simulink model "px4_6dof_quadrotor_simscape"  (R2023a)
settings: Solver=FixedStepAuto  StartTime=0.0  StopTime=timespot_spl(end)+2  FixedStep=0.001  MaxStep=1e-2  RelTol=1e-3  AbsTol=1e-3
model workspace (MATLAB code in the model file):
  | load('xy_data_membrane.mat');
undefined symbols (not defined in the file or in its folder): air_rho, battery_capacity, DiscIntNeverNeededParam, drone_leg, filtD_motor, filtSpd_motor, kd_motor, ki_motor, kp_motor, limit_motor, pkgSize, planedepth, qc_motor, qd_area, qd_drag, rad, s, spline_data, spline_yaw, timespot_spl, waypoints, wind_speed, X, Y, Z
libraries: sm_lib x77, nesl_utility x30, fl_lib x13, cstblocks x9, simulink x8, quadcopter_library x6, aerolibconvert2 x4, slpidlib x4, ee_lib x4, sharedtransform x1, batteryecm_lib x1
(part 1 of 4)
CloseFcn:
  | try,close(h1_quadcopter_package_delivery),end
  | clear h1_quadcopter_package_delivery
  | try,close(h2_quadcopter_package_delivery),end
  | clear h2_quadcopter_package_delivery
  | try,close(h3_quadcopter_package_delivery),end
  | clear h3_quadcopter_package_delivery
  | try,close(h4_quadcopter_package_delivery),end
  | clear h4_quadcopter_package_delivery
Description:
  | Quadcopter Package Delivery
  | Copyright 2021-2023 The MathWorks, Inc.
settings Model: VariantFading=off  Creator=tianwang  LastModifiedBy=user
settings SolverCC: AutoScaleAbsTol=off  AlgebraicLoopSolver=TrustRegion  SolverResetMethod=Robust
settings DataIOCC: MaxDataPoints=10000  ReturnWorkspaceOutputs=off  SignalLoggingName=logsout_quadcopter_package_delivery
settings OptimizationCC: ReuseModelBlockBuffer=off
settings DebuggingCC: ParameterPrecisionLossMsg=none  UnconnectedInputMsg=warning  UnconnectedOutputMsg=warning  UnconnectedLineMsg=warning
settings ModelReferenceCC: EnableRefExpFcnMdlSchedulingChecks=on
settings SFSimCC: CustomCodeUndefinedFunction=UseInterfaceOnly
settings RTWCC: DLArmComputeVersion=19.05
settings SimscapeCC: ExplicitSolverDiagnosticOptions=none  SimscapeLogType=all  SimscapeLogSimulationStatistics=on  SimscapeLogToSDI=on  SimscapeLogName=simlog_quadcopter_package_delivery  SimscapeLogLimitData=off  SimscapeLogDataHistory=50000
settings DiagnosticsConfigSet: SimMechanicsConflictingReferenceFrames=none  SimMechanicsRigidlyBoundBlock=none
settings ExplorerConfigSet: InternalSimMechanicsExplorerSettings="<ExplorerConfiguration><canonicalview>default</canonicalview><AnimationSetting><BasePlaybackSpeed>1.0</BasePlaybackSpeed><PlaybackSpeedFactor>2.0</PlaybackSpeedFactor></AnimationSetting><TilePanel><TileInfo><Tiles Columns=\"2\" Count=\"4\" Rows=\"2\"><Column Weight=\"0.5664\"/><Column Weight=\"0.4336\"/><Row Weight=\"0.3531\"/><Row Weight=\"0.6469\"/><Tile Height=\"1\" Width=\"1\" X=\"0\" Y=\"0\"/><Tile Height=\"1\" Width=\"1\" X=\"0\" Y=\"1\"/><Tile Height=\"1\" Width=\"1\" X=\"1\" Y=\"0\"/><Tile Height=\"1\" Width=\"1\" X=\"1\" Y=\"1\"/></Tiles></TileInfo><SceneInfo><SceneViewer><BGColor><R>1</R><G>1</G><B>1</B></BGColor><Camera><DoPerspective>off</DoPerspective><Position><X>3.00027489530859626</X><Y>2.64492473252887361</Y><Z>13.644244441979108</Z></Position><Center><X>3.00027489530859626</X><Y>2.64492473252887361</Y><Z>3.00000062058594352</Z></Center><Up><X>0</X><Y>1</Y><Z>-0</Z></Up><ViewLimDist>1</ViewLimDist><YLim>10.5985457420349132</YLim><XLim>33.4261827248793395</XLim></Camera></SceneViewer><SceneViewer><BGColor><R>1</R><G>1</G><B>1</B></BGColor><Camera><DoPerspective>on</DoPerspective><Position><X>5.02017998369651863</X><Y>7.98844218227809488</Y><Z>3.70518563279751856</Z></Position><Center><X>5.02017998369651863</X><Y>7.98844218227809488</Y><Z>2.70518563279751856</Z></Center><Up><X>0</X><Y>1</Y><Z>0</Z></Up><ViewLimDist>1</ViewLimDist><YLim>0.466307658154998583</YLim><XLim>0.796608916014789226</XLim></Camera></SceneViewer><SceneViewer><BGColor><R>1</R><G>1</G><B>1</B></BGColor><Camera><DoPerspective>on</DoPerspective><Position><X>6.5</X><Y>6.5</Y><Z>1</Z></Position><Center><X>5</X><Y>8</Y><Z>0</Z></Center><Up><X>0</X><Y>0</Y><Z>1</Z></Up><ViewLimDist>1</ViewLimDist><YLim>0.466307658154998583</YLim><XLim>1.12272536155780434</XLim></Camera></SceneViewer><SceneViewer><BGColor><R>1</R><G>1</G><B>1</B></BGColor><Camera><DoPerspective>on</DoPerspective><Position><X>5.52017998369651863</X><Y>6.98844218227809488</Y><Z>3.70518563279751856</Z></Position><Center><X>5.1868466503631856</X><Y>7.65510884894476185</Y><Z>3.0385189661308516</Z></Center><Up><X>-0.298142396999971915</X><Y>0.596284793999944052</Y><Z>0.745355992499929787</Z></Up><ViewLimDist>1</ViewLimDist><YLim>0.466307658154998583</YLim><XLim>0.608142904177144006</XLim></Camera></SceneViewer></SceneInfo></TilePanel><MechEditorPanel><Cameras><Camera><Id>Camera1</Id><Value><Name>FixO Top</Name><NativeCamera><PositionTrackingFeature>Quadcopter.Camera.Cam_FixO_Top.R</PositionTrackingFeature><CenterTrackingFeature>Quadcopter.Camera.Cam_FixO_Top.R</CenterTrackingFeature><UpVectorTrackingFeature>Quadcopter.Camera.Cam_FixO_Top.R</UpVectorTrackingFeature><CenterTrackingOrigin>off</CenterTrackingOrigin><CenterTrackingDirection>+X</CenterTrackingDirection><UpVectorTrackingDirection>+Y</UpVectorTrackingDirection></NativeCamera></Value></Camera><Camera><Id>Camera2</Id><Value><Name>FixO L</Name><NativeCamera><PositionTrackingFeature>Quadcopter.Camera.Cam_FixO_L.R</PositionTrackingFeature><CenterTrackingFeature>Quadcopter.Camera.Cam_FixO_L.R</CenterTrackingFeature><UpVectorTrackingFeature>Quadcopter.Camera.Cam_FixO_L.R</UpVectorTrackingFeature><CenterTrackingOrigin>off</CenterTrackingOrigin><CenterTrackingDirection>+X</CenterTrackingDirection><UpVectorTrackingDirection>+Z</UpVectorTrackingDirection></NativeCamera></Value></Camera><Camera><Id>Camera3</Id><Value><Name>FixO F</Name><NativeCamera><PositionTrackingFeature>Quadcopter.Camera.Cam_FixO_F.R</PositionTrackingFeature><CenterTrackingFeature>Quadcopter.Camera.Cam_FixO_F.R</CenterTrackingFeature><UpVectorTrackingFeature>Quadcopter.Camera.Cam_FixO_F.R</UpVectorTrackingFeature><CenterTrackingOrigin>off</CenterTrackingOrigin><CenterTrackingDirection>+X</CenterTrackingDirection><UpVectorTrackingDirection>+Z</UpVectorTrackingDirection></NativeCamera></Value></Camera><Camera><Id>Camera4</Id><Value><Name>FixO UFL</Name><NativeCamera><PositionTrackingFeature>Quadcopter.Camera.Cam_FixO_UFL.R</PositionTrackingFeature><CenterTrackingFeature>Quadcopter.Camera.Cam_FixO_UFL.R</CenterTrackingFeature><UpVectorTrackingFeature>Quadcopter.Camera.Cam_FixO_UFL.R</UpVectorTrackingFeature><CenterTrackingOrigin>off</CenterTrackingOrigin><CenterTrackingDirection>+X</CenterTrackingDirection><UpVectorTrackingDirection>+Z</UpVectorTrackingDirection></NativeCamera></Value></Camera><Camera><Id>Camera5</Id><Value><Name>Track_Target</Name><NativeCamera><PositionTrackingFeature>Quadcopter.Camera.Cam_Target.R</PositionTrackingFeature><CenterTrackingFeature>Quadcopter.Camera.Transform_Target.F</CenterTrackingFeature><UpVectorTrackingFeature>Quadcopter.Camera.Transform_Target.F</UpVectorTrackingFeature><CenterTrackingOrigin>on</CenterTrackingOrigin><UpVectorTrackingDirection>+Z</UpVectorTrackingDirection></NativeCamera></Value></Camera><Camera><Id>Camera6</Id><Value><Name>Track Body Forward</Name><NativeCamera><PositionTrackingFeature>Quadcopter.Body.Body.Cam_Body_Front.R</PositionTrackingFeature><CenterTrackingFeature>Quadcopter.Body.Body.Cam_Body_Front.R</CenterTrackingFeature><UpVectorTrackingFeature>Quadcopter.Body.Body.Cam_Body_Front.R</UpVectorTrackingFeature><CenterTrackingOrigin>off</CenterTrackingOrigin><CenterTrackingDirection>+X</CenterTrackingDirection><UpVectorTrackingDirection>+Z</UpVectorTrackingDirection></NativeCamera></Value></Camera></Cameras><GfxPanelCameraMap><MapElement CameraMLId=\"Camera1\" GfxPanelIndex=\"1\"/><MapElement CameraMLId=\"Camera5\" GfxPanelIndex=\"2\"/><MapElement CameraMLId=\"Camera4\" GfxPanelIndex=\"3\"/></GfxPanelCameraMap><VideoCreator><PlaybackSpeedRatio>1.0</PlaybackSpeedRatio><FrameRate>60</FrameRate><VideoFormat>MPEG-4</VideoFormat><FrameSize>[1920 1080]</FrameSize></VideoCreator></MechEditorPanel></ExplorerConfiguration>"

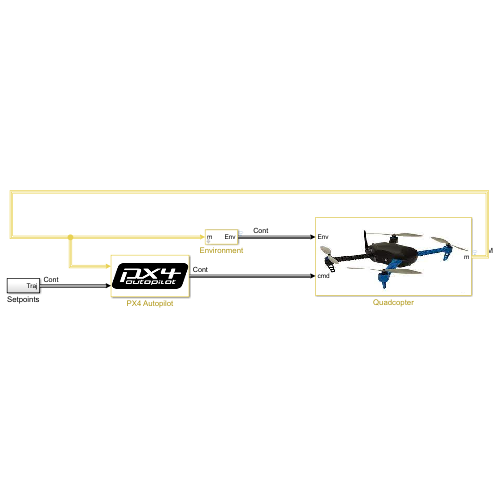
[thumbnail: Simulink's stored preview of the top-level diagram]
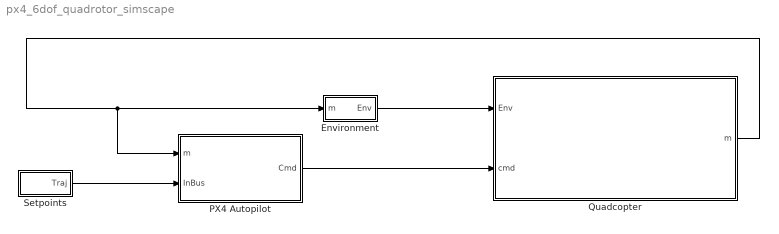
== system px4_6dof_quadrotor_simscape ==
  Environment : Subsystem  mask{wind_speed_mag=wind_speed, height_max_wind=6, height_min_wind=2}
      mask prompts: wind_speed_mag "Wind Speed for Gust (m/s)"; height_max_wind "Lowest Height for Max Wind (m)"; height_min_wind "Maximum Height for Zero Wind (m)"
  PX4 Autopilot : Subsystem
      mask Display:
      | image('C:\Users\user\Desktop\px4_simulink_simulator\docs\px4.png'); % Use "Edit Image" on toolstrip to change.
      | 
      | % port_label('input',1,'m')
      | % port_label('input',2,'Position S.P')
      | %
      | % port_label('output',1,'cmd','texmode','on')
  Quadcopter : Subsystem
      mask Display: image('C:\Users\user\Desktop\px4_simulink_simulator\docs\iris.jpg'); % Use "Edit Image" on toolstrip to change.
  Setpoints : Subsystem
  wires:
  Quadcopter/1(m) -> Environment/1(m), PX4 Autopilot/1(m)
  Setpoints/1(Traj) -> PX4 Autopilot/2(InBus)
  Environment/1(Env) -> Quadcopter/1(Env)
  PX4 Autopilot/1(Cmd) -> Quadcopter/2(cmd)

== system px4_6dof_quadrotor_simscape/Environment ==
  In Bus Element : Inport  PortName=m  Element=Chassis.pz
  Bias Height Min Wind : Bias  Bias=-height_min_wind  SaturateOnIntegerOverflow=off
  Bus Creator2 : BusCreator  Inputs=1
  Constant1 : Constant  Value=0
  Mux1 : Mux  Inputs=3
  Product1 : Product
  Pulse Generator2 : DiscretePulseGenerator  PulseType=Time based  Amplitude=wind_speed_mag  Period=10  PulseWidth=25  PhaseDelay=5
  Pulse Generator3 : DiscretePulseGenerator  PulseType=Time based  Amplitude=wind_speed_mag  Period=10  PulseWidth=25  PhaseDelay=9
  Saturation : Saturate  UpperLimit=height_max_wind-height_min_wind  LowerLimit=0  ZeroCross=off
  "Scale Wind by Height " : Gain  Gain=1/(height_max_wind-height_min_wind)
  Vec to Bus : Subsystem
  Env : Outport
  wires:
  In Bus Element/1 -> Bias Height Min Wind/1
  Bias Height Min Wind/1 -> Saturation/1
  Saturation/1 -> "Scale Wind by Height "/1
  "Scale Wind by Height "/1 -> Product1/1
  Constant1/1 -> Mux1/3  "vz"
  Pulse Generator3/1 -> Mux1/2  "vy"
  Pulse Generator2/1 -> Mux1/1  "vx"
  Mux1/1 -> Product1/2  "wind"
  Product1/1 -> Vec to Bus/1(V)  "wind"
  Vec to Bus/1(B) -> Bus Creator2/1
  Bus Creator2/1 -> Env/1  "Env"

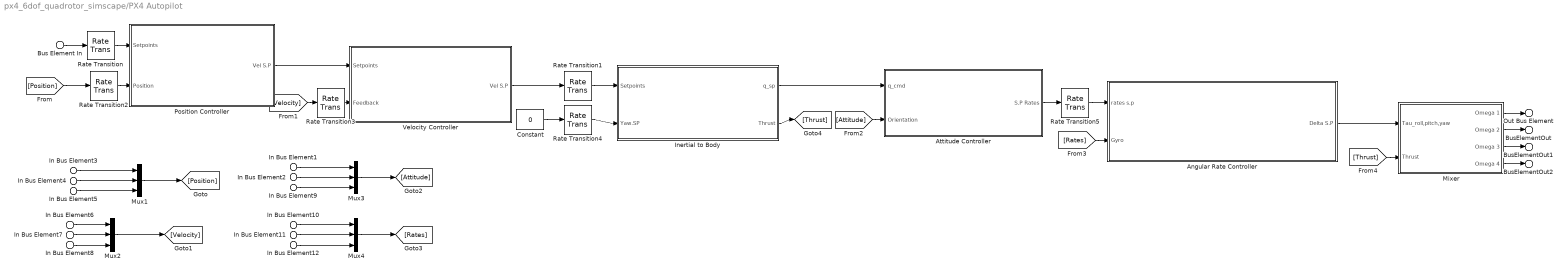
== system px4_6dof_quadrotor_simscape/PX4 Autopilot ==
  In Bus Element3 : Inport  PortName=m  Element=Chassis.px
  In Bus Element4 : Inport  PortName=m  Element=Chassis.py
  In Bus Element5 : Inport  PortName=m  Element=Chassis.pz
  In Bus Element6 : Inport  PortName=m  Element=Chassis.vx
  In Bus Element7 : Inport  PortName=m  Element=Chassis.vy
  In Bus Element8 : Inport  PortName=m  Element=Chassis.vz
  In Bus Element1 : Inport  PortName=m  Element=Chassis.roll
  In Bus Element2 : Inport  PortName=m  Element=Chassis.pitch
  In Bus Element9 : Inport  PortName=m  Element=Chassis.yaw
  In Bus Element10 : Inport  PortName=m  Element=Chassis.nRoll
  In Bus Element11 : Inport  PortName=m  Element=Chassis.nPitch
  In Bus Element12 : Inport  PortName=m  Element=Chassis.nYaw
  Bus Element In : Inport  Port=2  PortName=InBus  Element=pos
  Angular Rate Controller : Subsystem  mask{MC_ROLLRATE_K=1, MC_ROLLRATE_P=0.044, MC_ROLLRATE_I=0.05, MC_ROLLRATE_D=0.0012, MC_RR_INT_LIM=101, MC_PITCHRATE_K=1, MC_PITCHRATE_P=0.044, MC_PITCHRATE_I=0.05, MC_PITCHRATE_D=0.0012, MC_PR_INT_LIM=100, MC_YAWRATE_K=1, MC_YAWRATE_P=0.044, MC_YAWRATE_I=0.05, MC_YAWRATE_D=0.0012, MC_YR_INT_LIM=100, IMU_DGYRO_CUTOFF=6000, IMU_GYRO_CUTOFF=0}
      mask prompts: MC_ROLLRATE_K "MC_ROLLRATE_K ="; MC_ROLLRATE_P "MC_ROLLRATE_P ="; MC_ROLLRATE_I "MC_ROLLRATE_I ="; MC_ROLLRATE_D "MC_ROLLRATE_D ="; MC_RR_INT_LIM "MC_RR_INT_LIM ="; MC_PITCHRATE_K "MC_PITCHRATE_K ="; MC_PITCHRATE_P "MC_PITCHRATE_P ="; MC_PITCHRATE_I "MC_PITCHRATE_I ="; MC_PITCHRATE_D "MC_PITCHRATE_D ="; MC_PR_INT_LIM "MC_PR_INT_LIM ="; MC_YAWRATE_K "MC_YAWRATE_K ="; MC_YAWRATE_P "MC_YAWRATE_P ="; MC_YAWRATE_I "MC_YAWRATE_I ="; MC_YAWRATE_D "MC_YAWRATE_D ="; MC_YR_INT_LIM "MC_YR_INT_LIM ="; IMU_DGYRO_CUTOFF "IMU_DGYRO_CUTOFF ="; IMU_GYRO_CUTOFF "IMU_GYRO_CUTOFF ="
      mask DialogControl DescTextVar Prompt: Angular rate controller, based on PX4 architecture
      mask DialogControl ROLL Prompt: Roll
      mask DialogControl PITCH Prompt: Pitch
      mask DialogControl YAW Prompt: Yaw
      mask Display:
      | disp('Angular Rate Controller')
      | 
      | port_label('input',1,'RATE S.P','texmode','on')
      | port_label('input',2,'Rates','texmode','on')
      | 
      | port_label('output',1,'\delta_{cmd}','texmode','on')
  Attitude Controller : Subsystem  mask{MC_ROLL_P=4, MC_PITCH_P=4, MC_YAW_P=4, MC_ROLLRATE_MAX=2, MC_PITCHRATE_MAX=2, MC_YAWRATE_MAX=2, MC_ACRO_R_MAX=2, MC_YAW_WEIGHT=0.1, m=0.9}
      mask prompts: MC_ROLL_P "MC_ROLL_P ="; MC_PITCH_P "MC_PITCH_P ="; MC_YAW_P "MC_YAW_P ="; MC_ROLLRATE_MAX "MC_ROLLRATE_MAX ="; MC_PITCHRATE_MAX "MC_PITCHRATE_MAX ="; MC_YAWRATE_MAX "MC_YAWRATE_MAX ="; MC_ACRO_R_MAX "MC_ACRO_R_MAX ="; MC_YAW_WEIGHT "MC_YAW_WEIGHT ="; m "m [kg] ="
      mask DialogControl DescTextVar Prompt: Attitude Controller - based on PX4 architecture
      mask Display:
      | disp('Attitude Controller')
      | 
      | port_label('input',1,'q_{sp}','texmode','on')
      | port_label('input',2,'Attitude')
      | 
      | port_label('output',1,'RATES S.P','texmode','on')
  Constant : Constant  Value=0
  Inertial to Body : Subsystem
      mask DialogControl DescTextVar Prompt: Attitude Controller - based on PX4 architecture
      mask Display:
      | disp('Inertial to Body')
      | 
      | port_label('input',1,'ACCEL. S.P')
      | port_label('input',2,'\psi_{cmd}','texmode','on')
      | 
      | port_label('output',1,'q_{sp}','texmode','on')
      | port_label('output',2,'Thrust_{cmd}','texmode','on')
  Mixer : Subsystem  mask{Ct=7e-6, Cq=1.6e-7, d=0.165}
      mask prompts: Ct "Ct ="; Cq "Cq ="; d "d [m] ="
      mask Display:
      | disp('Mixer')
      | 
      | port_label('input',1,'\delta_{cmd}','texmode','on')
      | port_label('input',2,'Thrust_{cmd}','texmode','on')
      | 
      | port_label('output',1,'\Omega_{1cmd}','texmode','on')
      | port_label('output',2,'\Omega_{2cmd}','texmode','on')
      | port_label('output',3,'\Omega_{3cmd}','texmode','on')
      | port_label('output',4,'\Omega_{4cmd}','texmode','on')
  Mux{1..4} (4 alike) : Mux  Inputs=3
  Position Controller : Subsystem  mask{MPC_XY_P=1, MPC_XY_VEL_MAX=10, MPC_Z_P=1, MPC_Z_VEL_MAX_UP=100, MPC_Z_VEL_MAX_DOWN=-100}
      mask prompts: MPC_XY_P "MPC_XY_P ="; MPC_XY_VEL_MAX "MPC_XY_VEL_MAX ="; MPC_Z_P "MPC_Z_P ="; MPC_Z_VEL_MAX_UP "MPC_Z_VEL_MAX_UP ="; MPC_Z_VEL_MAX_DOWN "MPC_Z_VEL_MAX_DOWN ="
      mask DialogControl DescTextVar Prompt: Position Controller - based on PX4 architecture
      mask Display:
      | disp('Position Controller')
      | 
      | port_label('input',1,'POS. S.P')
      | port_label('input',2,'Position')
      | 
      | port_label('output',1,'VEL. S.P','texmode','on')
  Rate Transition : RateTransition  OutPortSampleTime=1/50
  Rate Transition1 : RateTransition  OutPortSampleTime=1/1000
  Rate Transition2 : RateTransition  OutPortSampleTime=1/50
  Rate Transition3 : RateTransition  OutPortSampleTime=1/50
  Rate Transition4 : RateTransition  OutPortSampleTime=1/ 250
  Rate Transition5 : RateTransition  OutPortSampleTime=1/1000
  Velocity Controller : Subsystem  mask{MPC_XY_VEL_P_ACC=1, MPC_XY_VEL_I_ACC=0.1, MPC_XY_VEL_D_ACC=0.05, MPC_Z_VEL_P_ACC=1, MPC_Z_VEL_I_ACC=0.1, MPC_Z_VEL_D_ACC=0.05, MPC_VELD_LP=0, MPC_TILTMAX_AIR=1000, MPC_THR_MAX=10000}
      mask prompts: MPC_XY_VEL_P_ACC "MPC_XY_VEL_P_ACC ="; MPC_XY_VEL_I_ACC "MPC_XY_VEL_I_ACC ="; MPC_XY_VEL_D_ACC "MPC_XY_VEL_D_ACC ="; MPC_Z_VEL_P_ACC "MPC_Z_VEL_P_ACC ="; MPC_Z_VEL_I_ACC "MPC_Z_VEL_I_ACC ="; MPC_Z_VEL_D_ACC "MPC_Z_VEL_D_ACC ="; MPC_VELD_LP "MPC_VELD_LP ="; MPC_TILTMAX_AIR "MPC_TILTMAX_AIR ="; MPC_THR_MAX "MPC_THR_MAX ="
      mask DialogControl DescTextVar Prompt: Velocity Controller - based on PX4 architecture
      mask DialogControl Container3 Prompt: XY -  Velocity
      mask DialogControl Container4 Prompt: Z - Velocity
      mask DialogControl Container5 Prompt: General Parameters
      mask Display:
      | disp('Velocity Controller')
      | 
      | port_label('input',1,'VEL. S.P')
      | port_label('input',2,'Velocity')
      | 
      | port_label('output',1,'ACCEL. S.P','texmode','on')
  Out Bus Element : Outport  PortName=Cmd  Element=w1
  BusElementOut : Outport  PortName=Cmd  Element=w2
  BusElementOut1 : Outport  PortName=Cmd  Element=w3
  BusElementOut2 : Outport  PortName=Cmd  Element=w4
  wires:
  Inertial to Body/1(q_sp) -> Attitude Controller/1(q_cmd)
  Angular Rate Controller/1(Delta S.P) -> Mixer/1(Tau_roll,pitch,yaw)
  Rate Transition4/1 -> Inertial to Body/2(Yaw.SP)
  Velocity Controller/1(Vel S.P) -> Rate Transition1/1
  [Velocity] -> Rate Transition3/1
  Attitude Controller/1(S.P Rates) -> Rate Transition5/1
  Rate Transition5/1 -> Angular Rate Controller/1(rates s.p)
  Constant/1 -> Rate Transition4/1
  Mixer/1(Omega 1) -> Out Bus Element/1
  Mixer/2(Omega 2) -> BusElementOut/1
  Mixer/3(Omega 3) -> BusElementOut1/1
  Mixer/4(Omega 4) -> BusElementOut2/1
  In Bus Element5/1 -> Mux1/3
  In Bus Element4/1 -> Mux1/2
  In Bus Element3/1 -> Mux1/1
  [Position] -> Rate Transition2/1
  Position Controller/1(Vel S.P) -> Velocity Controller/1(Setpoints)
  In Bus Element8/1 -> Mux2/3
  In Bus Element6/1 -> Mux2/1
  In Bus Element7/1 -> Mux2/2
  [Attitude] -> Attitude Controller/2(Orientation)
  In Bus Element9/1 -> Mux3/3
  In Bus Element1/1 -> Mux3/1
  In Bus Element2/1 -> Mux3/2
  Bus Element In/1 -> Rate Transition/1
  Rate Transition1/1 -> Inertial to Body/1(Setpoints)
  [Rates] -> Angular Rate Controller/2(Gyro)
  In Bus Element10/1 -> Mux4/1
  In Bus Element12/1 -> Mux4/3
  In Bus Element11/1 -> Mux4/2
  Mux1/1 -> [Position]
  Mux2/1 -> [Velocity]
  Mux3/1 -> [Attitude]
  Mux4/1 -> [Rates]
  Inertial to Body/2(Thrust) -> [Thrust]
  [Thrust] -> Mixer/2(Thrust)
  Rate Transition/1 -> Position Controller/1(Setpoints)
  Rate Transition2/1 -> Position Controller/2(Position)
  Rate Transition3/1 -> Velocity Controller/2(Feedback)

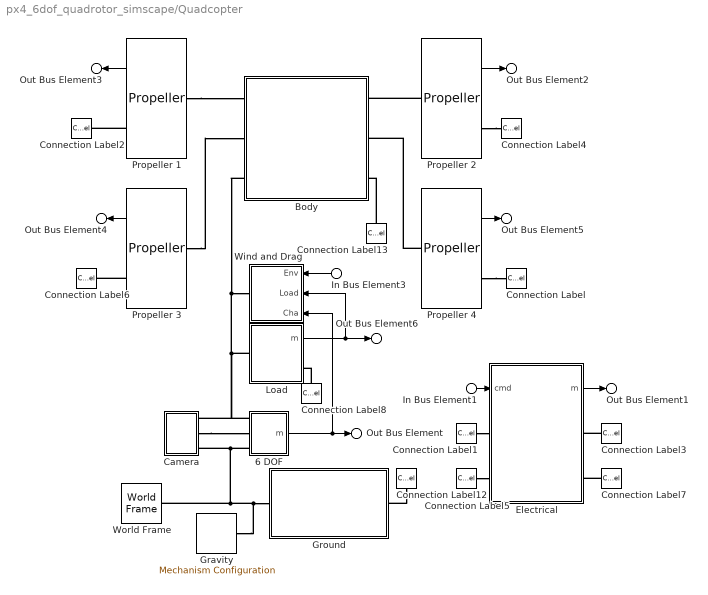
== system px4_6dof_quadrotor_simscape/Quadcopter ==
  In Bus Element3 : Inport  PortName=Env  Element=wind
  In Bus Element1 : Inport  Port=2  PortName=cmd
  6 DOF : Subsystem
  Body : Subsystem
      mask Display: image('quadcopter_body_arms.png');
  Camera : Subsystem
  Connection Label : ConnectionLabel  Label=P4
  Connection Label1 : ConnectionLabel  Label=P4
  Connection Label12 : ConnectionLabel  Label=G
  Connection Label13 : ConnectionLabel  Label=G
  Connection Label2 : ConnectionLabel  Label=P1
  Connection Label3 : ConnectionLabel  Label=P1
  Connection Label4 : ConnectionLabel  Label=P2
  Connection Label5 : ConnectionLabel  Label=P2
  Connection Label6 : ConnectionLabel  Label=P3
  Connection Label7 : ConnectionLabel  Label=P3
  Connection Label8 : ConnectionLabel  Label=G
  Electrical : Subsystem  mask{trq_max=qc_motor.max_torque, power_max=qc_motor.max_power, trq_tc=qc_motor.time_const, eff_overall=qc_motor.efficiency, eff_spd=qc_motor.efficiency_spd, eff_trq=qc_motor.efficiency_trq, rotor_d=qc_motor.rotor_damping, kp=kp_motor, ki=ki_motor, kd=kd_motor, f_deriv=filtD_motor, f_spd=filtSpd_motor, max_trq_cmd=limit_motor}
      mask prompts: trq_max "Max Torque (N*m)"; power_max "Max Power (W)"; trq_tc "Time Constant, Torque (s)"; eff_overall "Efficiency (%)"; eff_spd "Speed for Efficiency (rpm)"; eff_trq "Torque for Efficiency (N*m)"; rotor_d "Rotor Damping (N*m/(rad/s))"; kp "Proportional"; ki "Integral"; kd "Derivative"; f_deriv "Filter on Error Derivative (N)"; f_spd "Filter on Speed Measurement (sec)"; max_trq_cmd "Saturation (N*m)"
      mask DialogControl Container4 Prompt: Motor
      mask DialogControl Container9 Prompt: Control
      mask Display: image('quadcopter_electric.png');
  Gravity : sm_lib/Utilities/Mechanism Configuration  UniformGravity=Constant  GravityVector=[0 0 -9.80665]  GravityVectorUnits=m/s^2  LinearizationDelta=0.001  JointModeTransitionNonlinearIterations=2
  Ground : Subsystem
      mask Display: image('ground_launch_target.PNG');
  Load : Subsystem
      mask Display:
      | %image('medical_kit.png');
      | image('load_package_basket.png');
  Propeller 1 : quadcopter_library/Propeller  popup_prop_pos=1 or 4
  Propeller 2 : quadcopter_library/Propeller  popup_prop_pos=2 or 3
  Propeller 3 : quadcopter_library/Propeller  popup_prop_pos=2 or 3
  Propeller 4 : quadcopter_library/Propeller  popup_prop_pos=1 or 4
  Wind and Drag : Subsystem
  World Frame : sm_lib/Frames and Transforms/World Frame
  Out Bus Element : Outport  PortName=m  Element=Chassis
  Out Bus Element1 : Outport  PortName=m  Element=Motor
  Out Bus Element2 : Outport  PortName=m  Element=Prop2
  Out Bus Element3 : Outport  PortName=m  Element=Prop1
  Out Bus Element4 : Outport  PortName=m  Element=Prop3
  Out Bus Element5 : Outport  PortName=m  Element=Prop4
  Out Bus Element6 : Outport  PortName=m  Element=Load
  wires:
  Propeller 4/1 -> Out Bus Element5/1
  Propeller 1/1 -> Out Bus Element3/1
  Propeller 3/1 -> Out Bus Element4/1
  Electrical/1(m) -> Out Bus Element1/1
  Propeller 2/1 -> Out Bus Element2/1
  In Bus Element1/1 -> Electrical/1(cmd)
  6 DOF/1(m) -> Out Bus Element/1, Wind and Drag/3(Cha)
  Load/1(m) -> Out Bus Element6/1, Wind and Drag/2(Load)
  In Bus Element3/1 -> Wind and Drag/1(Env)
  connections:
  Body/LConn3 -- 6 DOF/LConn1 -- Camera/RConn1 -- Load/LConn1 -- Wind and Drag/RConn1
  Propeller 2/LConn1 -- Body/RConn1
  Propeller 1/LConn1 -- Body/LConn1
  Propeller 4/LConn1 -- Body/RConn2
  Propeller 3/LConn1 -- Body/LConn2
  Connection Label13/LConn1 -- Body/RConn3
  Propeller 4/RConn1 -- Connection Label/LConn1
  Connection Label1/LConn1 -- Electrical/LConn1
  Propeller 1/RConn1 -- Connection Label2/LConn1
  Connection Label3/LConn1 -- Electrical/RConn1
  Propeller 2/RConn1 -- Connection Label4/LConn1
  Connection Label5/LConn1 -- Electrical/LConn2
  Propeller 3/RConn1 -- Connection Label6/LConn1
  Connection Label7/LConn1 -- Electrical/RConn2
  Gravity/RConn1 -- 6 DOF/LConn3 -- Camera/RConn3 -- World Frame/RConn1 -- Ground/RConn1
  Connection Label12/LConn1 -- Ground/LConn1
  Connection Label8/LConn1 -- Load/RConn1
  Camera/RConn2 -- 6 DOF/LConn2

== system px4_6dof_quadrotor_simscape/Setpoints ==
  Clock1 : Clock
  Derivative : Subsystem
  Interpolate Spline Points : Subsystem
  Out Bus Element : Outport  PortName=Traj  Element=pos
  Out Bus Element1 : Outport  PortName=Traj  Element=vel
  Out Bus Element2 : Outport  PortName=Traj  Element=yaw
  wires:
  Clock1/1 -> Interpolate Spline Points/1(In1)
  Interpolate Spline Points/2(des_pos) -> Out Bus Element/1, Derivative/1(des xyz)
  Interpolate Spline Points/1(Yaw) -> Out Bus Element2/1
  Derivative/1(des_vel) -> Out Bus Element1/1

== system px4_6dof_quadrotor_simscape/Environment/Vec to Bus ==
  V : Inport
  Bus Creator : BusCreator  Inputs=3
  Demux : Demux  Outputs=3
  B : Outport
  wires:
  Demux/3 -> Bus Creator/3  "vz"
  V/1 -> Demux/1
  Demux/1 -> Bus Creator/1  "vx"
  Demux/2 -> Bus Creator/2  "vy"
  Bus Creator/1 -> B/1  "wind"

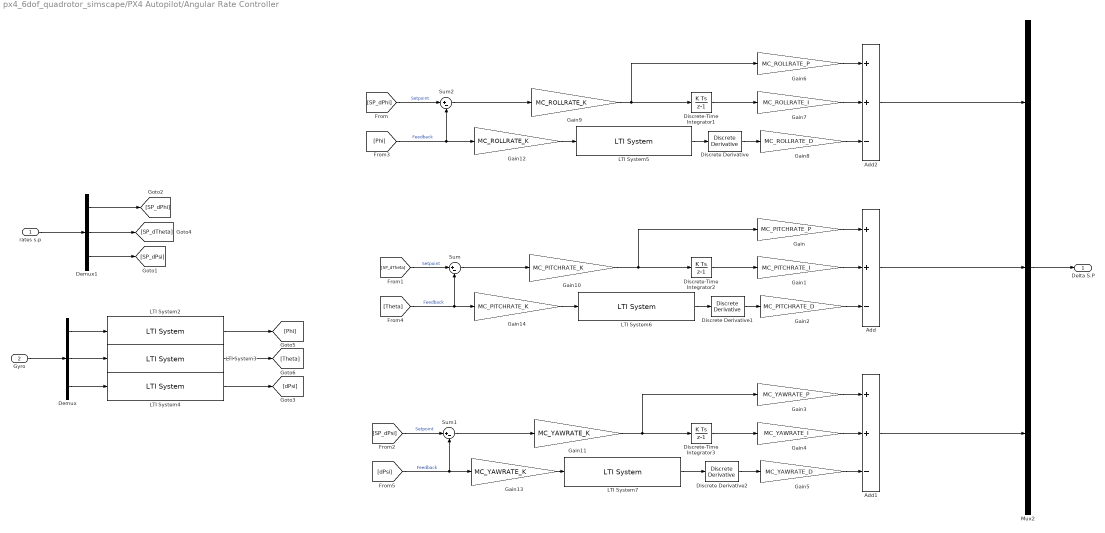
== system px4_6dof_quadrotor_simscape/PX4 Autopilot/Angular Rate Controller ==
  rates s.p : Inport
  Gyro : Inport  Port=2
  Add : Sum  Inputs=++-
  Add1 : Sum  Inputs=++-
  Add2 : Sum  Inputs=++-
  Demux : Demux  Outputs=3
  Demux1 : Demux  Outputs=3
  Discrete Derivative : simulink/Discrete/Discrete Derivative  gainval=1.0  ICPrevScaledInput=0.0  OutMin=[]  OutMax=[]  OutDataType=fixdt(1, 16)  OutScaling=2^-10  DoSatur=off
  Discrete Derivative1 : simulink/Discrete/Discrete Derivative  gainval=1.0  ICPrevScaledInput=0.0  OutMin=[]  OutMax=[]  OutDataType=fixdt(1, 16)  OutScaling=2^-10  DoSatur=off
  Discrete Derivative2 : simulink/Discrete/Discrete Derivative  gainval=1.0  ICPrevScaledInput=0.0  OutMin=[]  OutMax=[]  OutDataType=fixdt(1, 16)  OutScaling=2^-10  DoSatur=off
  Discrete-Time Integrator1 : DiscreteIntegrator  SampleTime=1/1000  LimitOutput=on  UpperSaturationLimit=MC_RR_INT_LIM  LowerSaturationLimit=-MC_RR_INT_LIM  ICPrevOutput=DiscIntNeverNeededParam  ICPrevScaledInput=DiscIntNeverNeededParam
  Discrete-Time Integrator2 : DiscreteIntegrator  SampleTime=1/1000  LimitOutput=on  UpperSaturationLimit=MC_PR_INT_LIM  LowerSaturationLimit=-MC_PR_INT_LIM  ICPrevOutput=DiscIntNeverNeededParam  ICPrevScaledInput=DiscIntNeverNeededParam
  Discrete-Time Integrator3 : DiscreteIntegrator  SampleTime=1/1000  LimitOutput=on  UpperSaturationLimit=MC_YR_INT_LIM  LowerSaturationLimit=-MC_YR_INT_LIM  ICPrevOutput=DiscIntNeverNeededParam  ICPrevScaledInput=DiscIntNeverNeededParam
  Gain : Gain  Gain=MC_PITCHRATE_P
  Gain1 : Gain  Gain=MC_PITCHRATE_I
  Gain10 : Gain  Gain=MC_PITCHRATE_K
  Gain11 : Gain  Gain=MC_YAWRATE_K
  Gain12 : Gain  Gain=MC_ROLLRATE_K
  Gain13 : Gain  Gain=MC_YAWRATE_K
  Gain14 : Gain  Gain=MC_PITCHRATE_K
  Gain2 : Gain  Gain=MC_PITCHRATE_D
  Gain3 : Gain  Gain=MC_YAWRATE_P
  Gain4 : Gain  Gain=MC_YAWRATE_I
  Gain5 : Gain  Gain=MC_YAWRATE_D
  Gain6 : Gain  Gain=MC_ROLLRATE_P
  Gain7 : Gain  Gain=MC_ROLLRATE_I
  Gain8 : Gain  Gain=MC_ROLLRATE_D
  Gain9 : Gain  Gain=MC_ROLLRATE_K
  LTI System2 : cstblocks/LTI System  sys=c2d(tf(1,[IMU_GYRO_CUTOFF 1]),1/1000)  IC=[]
  LTI System3 : cstblocks/LTI System  sys=c2d(tf(1,[IMU_GYRO_CUTOFF 1]),1/1000)  IC=[]
  LTI System4 : cstblocks/LTI System  sys=c2d(tf(1,[IMU_GYRO_CUTOFF 1]),1/1000)  IC=[]
  LTI System5 : cstblocks/LTI System  sys=c2d(tf(1,[IMU_DGYRO_CUTOFF 1]),1/1000)  IC=[]
  LTI System6 : cstblocks/LTI System  sys=c2d(tf(1,[IMU_DGYRO_CUTOFF 1]),1/1000)  IC=[]
  LTI System7 : cstblocks/LTI System  sys=c2d(tf(1,[IMU_DGYRO_CUTOFF 1]),1/1000)  IC=[]
  Mux2 : Mux  Inputs=3
  Sum : Sum  Inputs=|+-
  Sum1 : Sum  Inputs=|+-
  Sum2 : Sum  Inputs=|+-
  Delta S.P : Outport
  wires:
  LTI System6/1 -> Discrete Derivative1/1
  Sum/1 -> Gain10/1
  Discrete-Time Integrator2/1 -> Gain1/1
  Gain2/1 -> Add/3
  Gain1/1 -> Add/2
  Gain/1 -> Add/1
  Gain3/1 -> Add1/1
  Gain4/1 -> Add1/2
  Gain5/1 -> Add1/3
  Discrete-Time Integrator3/1 -> Gain4/1
  Sum1/1 -> Gain11/1
  LTI System7/1 -> Discrete Derivative2/1
  [dPsi] -> Gain13/1, Sum1/2  "Feedback"
  [SP_dPsi] -> Sum1/1  "Setpoint"
  Add/1 -> Mux2/2
  Mux2/1 -> Delta S.P/1
  Gain6/1 -> Add2/1
  Gain7/1 -> Add2/2
  Gain8/1 -> Add2/3
  Discrete-Time Integrator1/1 -> Gain7/1
  Sum2/1 -> Gain9/1
  LTI System5/1 -> Discrete Derivative/1
  [SP_dPhi] -> Sum2/1  "Setpoint"
  [SP_dTheta] -> Sum/1  "Setpoint"
  [Phi] -> Gain12/1, Sum2/2  "Feedback"
  [Theta] -> Gain14/1, Sum/2  "Feedback"
  Add1/1 -> Mux2/3
  Discrete Derivative/1 -> Gain8/1
  Discrete Derivative1/1 -> Gain2/1
  Discrete Derivative2/1 -> Gain5/1
  Gain9/1 -> Discrete-Time Integrator1/1, Gain6/1
  Gain10/1 -> Discrete-Time Integrator2/1, Gain/1
  Gain11/1 -> Discrete-Time Integrator3/1, Gain3/1
  Gain12/1 -> LTI System5/1
  Gain13/1 -> LTI System7/1
  Gain14/1 -> LTI System6/1
  Gyro/1 -> Demux/1
  Demux/1 -> LTI System2/1
  Demux/2 -> LTI System3/1
  Demux/3 -> LTI System4/1
  LTI System2/1 -> [Phi]
  LTI System3/1 -> [Theta]
  LTI System4/1 -> [dPsi]
  Add2/1 -> Mux2/1
  rates s.p/1 -> Demux1/1
  Demux1/1 -> [SP_dPhi]
  Demux1/2 -> [SP_dTheta]
  Demux1/3 -> [SP_dPsi]

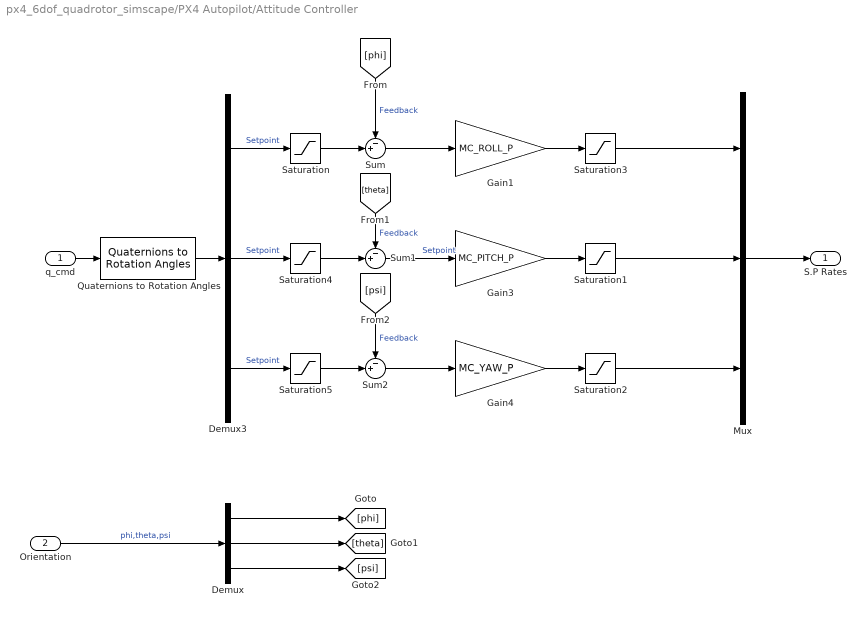
== system px4_6dof_quadrotor_simscape/PX4 Autopilot/Attitude Controller ==
  q_cmd : Inport
  Orientation : Inport  Port=2
  Demux : Demux  Outputs=3
  Demux3 : Demux  Outputs=3
  Gain1 : Gain  Gain=MC_ROLL_P
  Gain3 : Gain  Gain=MC_PITCH_P
  Gain4 : Gain  Gain=MC_YAW_P
  Mux : Mux  Inputs=3
  Quaternions to Rotation Angles : sharedtransform/Quaternions to Rotation Angles  rotationOrder=XYZ  aMode=aMode
  Saturation : Saturate  UpperLimit=1.5  LowerLimit=-1.5
  Saturation1 : Saturate  UpperLimit=MC_PITCHRATE_MAX  LowerLimit=-MC_PITCHRATE_MAX
  Saturation2 : Saturate  UpperLimit=MC_YAWRATE_MAX  LowerLimit=-MC_YAWRATE_MAX
  Saturation3 : Saturate  UpperLimit=MC_ROLLRATE_MAX  LowerLimit=-MC_ROLLRATE_MAX
  Saturation4 : Saturate  UpperLimit=1.5  LowerLimit=-1.5
  Saturation5 : Saturate  UpperLimit=1.5  LowerLimit=-1.5
  Sum : Sum  Inputs=-+|
  Sum1 : Sum  Inputs=-+|
  Sum2 : Sum  Inputs=-+|
  S.P Rates : Outport
  wires:
  Orientation/1 -> Demux/1  "phi,theta,psi"
  Demux/2 -> [theta]
  Demux/1 -> [phi]
  Demux/3 -> [psi]
  Demux3/1 -> Saturation/1  "Setpoint"
  Demux3/2 -> Saturation4/1  "Setpoint"
  Demux3/3 -> Saturation5/1  "Setpoint"
  Gain1/1 -> Saturation3/1
  Gain3/1 -> Saturation1/1
  Gain4/1 -> Saturation2/1
  Saturation1/1 -> Mux/2
  Saturation2/1 -> Mux/3
  [phi] -> Sum/1  "Feedback"
  Sum/1 -> Gain1/1
  [theta] -> Sum1/1  "Feedback"
  Sum2/1 -> Gain4/1
  [psi] -> Sum2/1  "Feedback"
  Sum1/1 -> Gain3/1  "Setpoint"
  q_cmd/1 -> Quaternions to Rotation Angles/1
  Quaternions to Rotation Angles/1 -> Demux3/1
  Saturation/1 -> Sum/2
  Saturation4/1 -> Sum1/2
  Saturation5/1 -> Sum2/2
  Saturation3/1 -> Mux/1
  Mux/1 -> S.P Rates/1

== system px4_6dof_quadrotor_simscape/PX4 Autopilot/Inertial to Body ==
  Setpoints : Inport
  Yaw.SP : Inport  Port=2
  Norm3 : Subsystem
      mask Display: disp('Norm')
  mass : Gain  Gain=1.0
  mavros attitude controller : Subsystem
      mask Display:
      | disp('Mavros Geometric controller')
      | port_label('input',1,'acc_{cmd}','texmode','on')
      | port_label('input',2,'\psi_{cmd}','texmode','on')
      | 
      | 
      | port_label('output',1,'quat','texmode','on')
  q_sp : Outport
  Thrust : Outport  Port=2
  wires:
  Norm3/1(Out1) -> mass/1
  mass/1 -> Thrust/1
  Yaw.SP/1 -> mavros attitude controller/2(yaw)
  mavros attitude controller/1(quat) -> q_sp/1
  Setpoints/1 -> mavros attitude controller/1(acc_cmd), Norm3/1(In1)

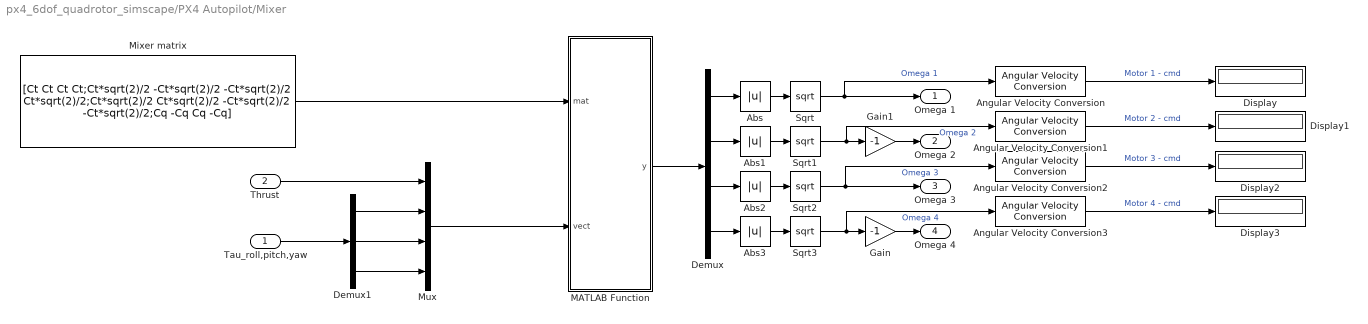
== system px4_6dof_quadrotor_simscape/PX4 Autopilot/Mixer ==
  Tau_roll,pitch,yaw : Inport
  Thrust : Inport  Port=2
  Abs{,1..3} (4 alike) : Abs  SaturateOnIntegerOverflow=off
  Angular Velocity Conversion{,1..3} (4 alike) : aerolibconvert2/Angular Velocity Conversion  IU=rad/s  OU=rpm
  Demux : Demux
  Demux1 : Demux  Outputs=3
  Display{,1..3} (4 alike) : Display
  Gain : Gain  Gain=-1
  Gain1 : Gain  Gain=-1
  MATLAB Function : MATLAB Function  TreatAsAtomicUnit=on
  Mixer matrix : Constant  StartFcn=|  Value=[Ct Ct Ct Ct;Ct*sqrt(2)/2 -Ct*sqrt(2)/2 -Ct*sqrt(2)/2 Ct*sqrt(2)/2;Ct*sqrt(2)/2 Ct*sqrt(2)/2 -Ct*sqrt(2)/2 -Ct*sqrt(2)/2;Cq -Cq Cq -Cq]  OutDataTypeStr=Inherit: Inherit via back propagation  SampleTime=1/1000
      | %p = Simulink.Mask.get('ControlsModels/Moments and Forces');
      | 
      | Ct = 0.025
      | Cq = 2e-6;
      | 
      | %Ct = p.getParameter('Ct');
      | %Cq =p.getParameter('Cq');
      | 
      | %Ct = str2double(Ct.Value);
      | %Cq = str2double(Cq.Value);
  Mux : Mux
  Sqrt{,1..3} (4 alike) : Sqrt
  Omega 1 : Outport
  Omega 2 : Outport  Port=2
  Omega 3 : Outport  Port=3
  Omega 4 : Outport  Port=4
  wires:
  Thrust/1 -> Mux/1
  Demux/1 -> Abs/1
  Demux/2 -> Abs1/1
  Demux/3 -> Abs2/1
  Demux/4 -> Abs3/1
  MATLAB Function/1(y) -> Demux/1
  Mux/1 -> MATLAB Function/2(vect)
  Mixer matrix/1 -> MATLAB Function/1(mat)
  Sqrt/1 -> Angular Velocity Conversion/1, Omega 1/1  "Omega 1"
  Sqrt1/1 -> Angular Velocity Conversion1/1, Gain1/1  "Omega 2"
  Sqrt2/1 -> Angular Velocity Conversion2/1, Omega 3/1  "Omega 3"
  Sqrt3/1 -> Angular Velocity Conversion3/1, Gain/1  "Omega 4"
  Tau_roll,pitch,yaw/1 -> Demux1/1
  Demux1/3 -> Mux/4
  Demux1/1 -> Mux/2
  Demux1/2 -> Mux/3
  Angular Velocity Conversion/1 -> Display/1  "Motor 1 - cmd"
  Angular Velocity Conversion1/1 -> Display1/1  "Motor 2 - cmd"
  Angular Velocity Conversion2/1 -> Display2/1  "Motor 3 - cmd"
  Angular Velocity Conversion3/1 -> Display3/1  "Motor 4 - cmd"
  Abs/1 -> Sqrt/1
  Abs1/1 -> Sqrt1/1
  Abs2/1 -> Sqrt2/1
  Abs3/1 -> Sqrt3/1
  Gain/1 -> Omega 4/1
  Gain1/1 -> Omega 2/1

== system px4_6dof_quadrotor_simscape/PX4 Autopilot/Position Controller ==
  Setpoints : Inport
  Position : Inport  Port=2
  Demux : Demux  Outputs=3
  Demux1 : Demux  Outputs=3
  Display : Display
  Gain : Gain  Gain=MPC_XY_P
  Gain1 : Gain  Gain=MPC_XY_P
  Gain2 : Gain  Gain=MPC_Z_P
  Mux : Mux  Inputs=3
  Saturation : Saturate  UpperLimit=MPC_XY_VEL_MAX  LowerLimit=-MPC_XY_VEL_MAX
  Saturation1 : Saturate  UpperLimit=MPC_XY_VEL_MAX  LowerLimit=-MPC_XY_VEL_MAX
  Saturation2 : Saturate  UpperLimit=MPC_Z_VEL_MAX_UP  LowerLimit=MPC_Z_VEL_MAX_DOWN
  Sum : Sum  Inputs=+-|
  Sum1 : Sum  Inputs=+-|
  Sum2 : Sum  Inputs=+-|
  Vel S.P : Outport
  wires:
  Demux/1 -> Sum/2  "x"
  Demux1/1 -> Sum/1  "sp_x"
  Demux/2 -> Sum1/2  "y"
  Demux1/2 -> Sum1/1  "sp_y"
  Demux/3 -> Sum2/2  "z"
  Demux1/3 -> Sum2/1  "sp_z"
  Sum/1 -> Gain/1
  Sum1/1 -> Gain1/1
  Sum2/1 -> Gain2/1
  Gain/1 -> Saturation/1
  Gain1/1 -> Saturation1/1
  Gain2/1 -> Saturation2/1
  Saturation2/1 -> Mux/3
  Saturation1/1 -> Mux/2
  Saturation/1 -> Mux/1
  Mux/1 -> Display/1, Vel S.P/1
  Position/1 -> Demux/1
  Setpoints/1 -> Demux1/1

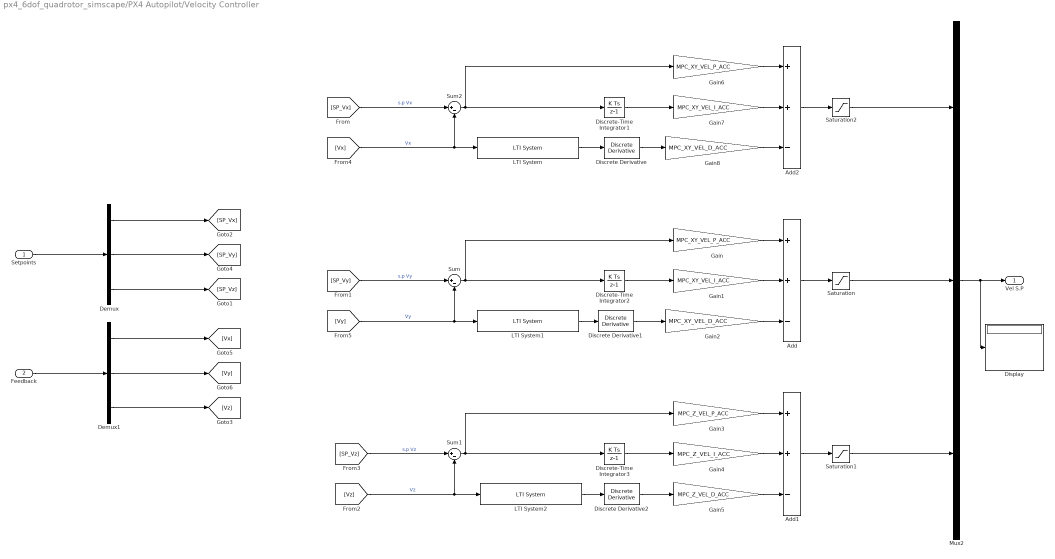
== system px4_6dof_quadrotor_simscape/PX4 Autopilot/Velocity Controller ==
  Setpoints : Inport
  Feedback : Inport  Port=2
  Add : Sum  Inputs=++-
  Add1 : Sum  Inputs=++-
  Add2 : Sum  Inputs=++-
  Demux : Demux  Outputs=3
  Demux1 : Demux  Outputs=3
  Discrete Derivative : simulink/Discrete/Discrete Derivative  gainval=1.0  ICPrevScaledInput=0.0  OutMin=[]  OutMax=[]  OutDataType=fixdt(1, 16)  OutScaling=2^-10  DoSatur=off
  Discrete Derivative1 : simulink/Discrete/Discrete Derivative  gainval=1.0  ICPrevScaledInput=0.0  OutMin=[]  OutMax=[]  OutDataType=fixdt(1, 16)  OutScaling=2^-10  DoSatur=off
  Discrete Derivative2 : simulink/Discrete/Discrete Derivative  gainval=1.0  ICPrevScaledInput=0.0  OutMin=[]  OutMax=[]  OutDataType=fixdt(1, 16)  OutScaling=2^-10  DoSatur=off
  Discrete-Time Integrator1 : DiscreteIntegrator  SampleTime=1/100  ICPrevOutput=DiscIntNeverNeededParam  ICPrevScaledInput=DiscIntNeverNeededParam
  Discrete-Time Integrator2 : DiscreteIntegrator  SampleTime=1/100  ICPrevOutput=DiscIntNeverNeededParam  ICPrevScaledInput=DiscIntNeverNeededParam
  Discrete-Time Integrator3 : DiscreteIntegrator  SampleTime=1/100  ICPrevOutput=DiscIntNeverNeededParam  ICPrevScaledInput=DiscIntNeverNeededParam
  Display : Display
  Gain : Gain  Gain=MPC_XY_VEL_P_ACC
  Gain1 : Gain  Gain=MPC_XY_VEL_I_ACC
  Gain2 : Gain  Gain=MPC_XY_VEL_D_ACC
  Gain3 : Gain  Gain=MPC_Z_VEL_P_ACC
  Gain4 : Gain  Gain=MPC_Z_VEL_I_ACC
  Gain5 : Gain  Gain=MPC_Z_VEL_D_ACC
  Gain6 : Gain  Gain=MPC_XY_VEL_P_ACC
  Gain7 : Gain  Gain=MPC_XY_VEL_I_ACC
  Gain8 : Gain  Gain=MPC_XY_VEL_D_ACC
  LTI System : cstblocks/LTI System  sys=c2d(tf(1,[MPC_VELD_LP 1]),1/100)  IC=[]
  LTI System1 : cstblocks/LTI System  sys=c2d(tf(1,[MPC_VELD_LP 1]),1/100)  IC=[]
  LTI System2 : cstblocks/LTI System  sys=c2d(tf(1,[MPC_VELD_LP 1]),1/100)  IC=[]
  Mux2 : Mux  Inputs=3
  Saturation : Saturate  UpperLimit=MPC_TILTMAX_AIR  LowerLimit=-MPC_TILTMAX_AIR
  Saturation1 : Saturate  UpperLimit=MPC_THR_MAX  LowerLimit=0
  Saturation2 : Saturate  UpperLimit=MPC_TILTMAX_AIR  LowerLimit=-MPC_TILTMAX_AIR
  Sum : Sum  Inputs=|+-
  Sum1 : Sum  Inputs=|+-
  Sum2 : Sum  Inputs=|+-
  Vel S.P : Outport
  wires:
  Setpoints/1 -> Demux/1
  Demux/3 -> [SP_Vz]
  Demux1/3 -> [Vz]
  Feedback/1 -> Demux1/1
  LTI System1/1 -> Discrete Derivative1/1
  Sum/1 -> Discrete-Time Integrator2/1, Gain/1
  Discrete-Time Integrator2/1 -> Gain1/1
  Gain2/1 -> Add/3
  Gain1/1 -> Add/2
  Gain/1 -> Add/1
  Add/1 -> Saturation/1
  Add1/1 -> Saturation1/1
  Gain3/1 -> Add1/1
  Gain4/1 -> Add1/2
  Gain5/1 -> Add1/3
  Discrete-Time Integrator3/1 -> Gain4/1
  Sum1/1 -> Discrete-Time Integrator3/1, Gain3/1
  LTI System2/1 -> Discrete Derivative2/1
  [Vz] -> LTI System2/1, Sum1/2  "Vz"
  [SP_Vz] -> Sum1/1  "s.p Vz"
  Saturation/1 -> Mux2/2
  Mux2/1 -> Display/1, Vel S.P/1
  Add2/1 -> Saturation2/1
  Gain6/1 -> Add2/1
  Gain7/1 -> Add2/2
  Gain8/1 -> Add2/3
  Discrete-Time Integrator1/1 -> Gain7/1
  Sum2/1 -> Discrete-Time Integrator1/1, Gain6/1
  LTI System/1 -> Discrete Derivative/1
  Demux/1 -> [SP_Vx]
  Demux/2 -> [SP_Vy]
  [SP_Vx] -> Sum2/1  "s.p Vx"
  [SP_Vy] -> Sum/1  "s.p Vy"
  Demux1/1 -> [Vx]
  [Vx] -> LTI System/1, Sum2/2  "Vx"
  Demux1/2 -> [Vy]
  [Vy] -> LTI System1/1, Sum/2  "Vy"
  Saturation2/1 -> Mux2/1
  Saturation1/1 -> Mux2/3
  Discrete Derivative/1 -> Gain8/1
  Discrete Derivative1/1 -> Gain2/1
  Discrete Derivative2/1 -> Gain5/1

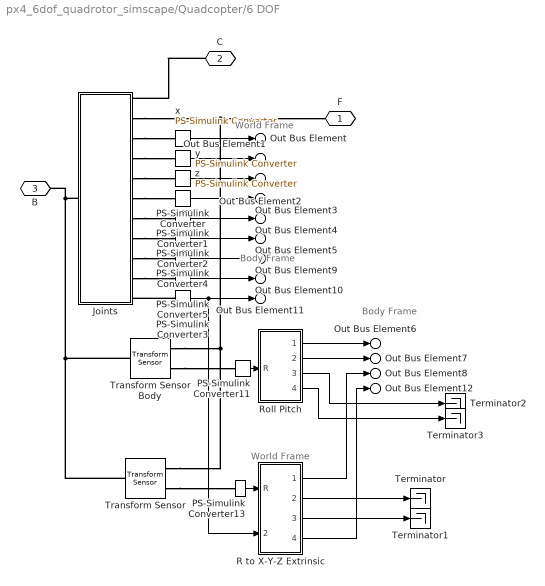
== system px4_6dof_quadrotor_simscape/Quadcopter/6 DOF ==
  note: Body Frame
  note: World Frame
  note: World Frame
  note: Body Frame
  Joints : Subsystem
  PS-Simulink Converter{,1..2,4..5} (5 alike) : nesl_utility/PS-Simulink Converter  PhysicalDomain=network_engine_domain  SubClassName=ps_output  LeftPortType=input  RightPortType=output  PseudoPeriodic=off  Frequencies=[]  VectorFormat=1-D array  Unit=inherit  AffineConversion=off
  PS-Simulink Converter11 : nesl_utility/PS-Simulink Converter  PhysicalDomain=network_engine_domain  SubClassName=ps_output  LeftPortType=input  RightPortType=output  PseudoPeriodic=off  Frequencies=[]  VectorFormat=1-D array  Unit=1  AffineConversion=off
  PS-Simulink Converter13 : nesl_utility/PS-Simulink Converter  PhysicalDomain=network_engine_domain  SubClassName=ps_output  LeftPortType=input  RightPortType=output  PseudoPeriodic=off  Frequencies=[]  VectorFormat=1-D array  Unit=1  AffineConversion=off
  PS-Simulink Converter3 : nesl_utility/PS-Simulink Converter  PhysicalDomain=network_engine_domain  SubClassName=ps_output  LeftPortType=input  RightPortType=output  PseudoPeriodic=off  Frequencies=[]  VectorFormat=1-D array  Unit=1  AffineConversion=off
  R to X-Y-Z Extrinsic : Subsystem  mask(Rotation Matrix to X-Y-Z Extrinsic){}
      mask help: Computes roll / pitch / yaw values assuming they correspond to X, Y, and Z rotations, applied in that order and using extrinsic rotations (rotations applied about the fixed axes of the base frame). Does not handle case where Y (pitch) rotation is +/-90 degrees.
  Roll Pitch : Subsystem
  Terminator{,1..3} (4 alike) : Terminator
  Transform Sensor : sm_lib/Frames and Transforms/Transform Sensor  MeasurementFrame=World  RotationSequence=XYX  SenseAngle=off  SenseAxis=off  SenseQ=off  SenseR=on  SenseRotationSequence=off  SenseOmegaX=off  SenseOmegaY=off  SenseOmegaZ=off  SenseQDot=off  SenseRDot=off  SenseRotationSequenceDot=off  SenseAlphaX=off  SenseAlphaY=off  SenseAlphaZ=off  SenseQDDot=off  SenseRDDot=off  SenseX=off  SenseY=off  SenseZ=off  SenseRad=off  SenseAzim=off  SenseDist=off  SenseInc=off  SenseXDot=off  SenseYDot=off  SenseZDot=off  SenseRadDot=off  SenseAzimDot=off  SenseDistDot=off  SenseIncDot=off  SenseXDDot=off  SenseYDDot=off  SenseZDDot=off  SenseRadDDot=off  SenseAzimDDot=off  SenseDistDDot=off  SenseIncDDot=off
  Transform Sensor Body : sm_lib/Frames and Transforms/Transform Sensor  MeasurementFrame=NonRotatingFollower  RotationSequence=XYX  SenseAngle=off  SenseAxis=off  SenseQ=off  SenseR=on  SenseRotationSequence=off  SenseOmegaX=off  SenseOmegaY=off  SenseOmegaZ=off  SenseQDot=off  SenseRDot=off  SenseRotationSequenceDot=off  SenseAlphaX=off  SenseAlphaY=off  SenseAlphaZ=off  SenseQDDot=off  SenseRDDot=off  SenseX=off  SenseY=off  SenseZ=off  SenseRad=off  SenseAzim=off  SenseDist=off  SenseInc=off  SenseXDot=off  SenseYDot=off  SenseZDot=off  SenseRadDot=off  SenseAzimDot=off  SenseDistDot=off  SenseIncDot=off  SenseXDDot=off  SenseYDDot=off  SenseZDDot=off  SenseRadDDot=off  SenseAzimDDot=off  SenseDistDDot=off  SenseIncDDot=off
  x : nesl_utility/PS-Simulink Converter  PhysicalDomain=network_engine_domain  SubClassName=ps_output  LeftPortType=input  RightPortType=output  PseudoPeriodic=off  Frequencies=[]  VectorFormat=1-D array  Unit=1  AffineConversion=off
  y : nesl_utility/PS-Simulink Converter  PhysicalDomain=network_engine_domain  SubClassName=ps_output  LeftPortType=input  RightPortType=output  PseudoPeriodic=off  Frequencies=[]  VectorFormat=1-D array  Unit=1  AffineConversion=off
  z : nesl_utility/PS-Simulink Converter  PhysicalDomain=network_engine_domain  SubClassName=ps_output  LeftPortType=input  RightPortType=output  PseudoPeriodic=off  Frequencies=[]  VectorFormat=1-D array  Unit=1  AffineConversion=off
  F : PMIOPort  Side=Left
  C : PMIOPort  Port=2  Side=Left
  B : PMIOPort  Port=3  Side=Left
  Out Bus Element : Outport  PortName=m  Element=px
  Out Bus Element1 : Outport  PortName=m  Element=vx
  Out Bus Element2 : Outport  PortName=m  Element=py
  Out Bus Element3 : Outport  PortName=m  Element=vy
  Out Bus Element4 : Outport  PortName=m  Element=pz
  Out Bus Element5 : Outport  PortName=m  Element=vz
  Out Bus Element6 : Outport  PortName=m  Element=roll
  Out Bus Element7 : Outport  PortName=m  Element=pitch
  Out Bus Element8 : Outport  PortName=m  Element=yaw
  Out Bus Element9 : Outport  PortName=m  Element=nRoll
  Out Bus Element10 : Outport  PortName=m  Element=nPitch
  Out Bus Element11 : Outport  PortName=m  Element=nYaw
  Out Bus Element12 : Outport  PortName=m  Element=yawWr
  wires:
  x/1 -> Out Bus Element/1
  y/1 -> Out Bus Element1/1
  R to X-Y-Z Extrinsic/1(yaw) -> Out Bus Element8/1
  PS-Simulink Converter1/1 -> Out Bus Element4/1
  PS-Simulink Converter2/1 -> Out Bus Element5/1
  z/1 -> Out Bus Element2/1
  PS-Simulink Converter/1 -> Out Bus Element3/1
  PS-Simulink Converter11/1 -> Roll Pitch/1(R)
  Roll Pitch/1(aRoll) -> Out Bus Element6/1
  Roll Pitch/2(aPitch) -> Out Bus Element7/1
  R to X-Y-Z Extrinsic/3(roll) -> Terminator1/1
  R to X-Y-Z Extrinsic/2(pitch) -> Terminator/1
  PS-Simulink Converter13/1 -> R to X-Y-Z Extrinsic/1(R)
  Roll Pitch/3(nRoll) -> Terminator2/1
  Roll Pitch/4(nPitch) -> Terminator3/1
  PS-Simulink Converter3/1 -> R to X-Y-Z Extrinsic/2(nYaw), Out Bus Element11/1
  PS-Simulink Converter4/1 -> Out Bus Element9/1
  PS-Simulink Converter5/1 -> Out Bus Element10/1
  R to X-Y-Z Extrinsic/4(yawWr) -> Out Bus Element12/1
  connections:
  Joints/RConn2 -- Transform Sensor/RConn1 -- Transform Sensor Body/RConn1 -- F/RConn1
  Joints/RConn3 -- x/LConn1
  Joints/RConn4 -- y/LConn1
  Transform Sensor Body/LConn1 -- Transform Sensor/LConn1 -- B/RConn1 -- Joints/LConn1
  Joints/RConn5 -- z/LConn1
  Joints/RConn6 -- PS-Simulink Converter/LConn1
  Joints/RConn7 -- PS-Simulink Converter1/LConn1
  Joints/RConn8 -- PS-Simulink Converter2/LConn1
  C/RConn1 -- Joints/RConn1
  Transform Sensor Body/RConn2 -- PS-Simulink Converter11/LConn1
  Transform Sensor/RConn2 -- PS-Simulink Converter13/LConn1
  PS-Simulink Converter3/LConn1 -- Joints/RConn11
  Joints/RConn9 -- PS-Simulink Converter4/LConn1
  Joints/RConn10 -- PS-Simulink Converter5/LConn1
